simulink model "faultdetectioninagrid"  (R2021a)
settings: Solver=VariableStepAuto  StartTime=0.0  StopTime=10.0  RelTol=1e-3
libraries: spsMosfetLib x20, spsSeriesRLCBranchLib x16, spsVoltageMeasurementLib x13, spsCurrentMeasurementLib x10, spsPiSectionLineLib x10, pid_lib x9, spsGroundLib x6, spsMeanLib x5, simulink x5, spsACVoltageSourceLib x4, spsPLLLib x4, spsDiodeLib x1
settings Model: Creator=Himanik Panchal  LastModifiedBy=Himanik Panchal

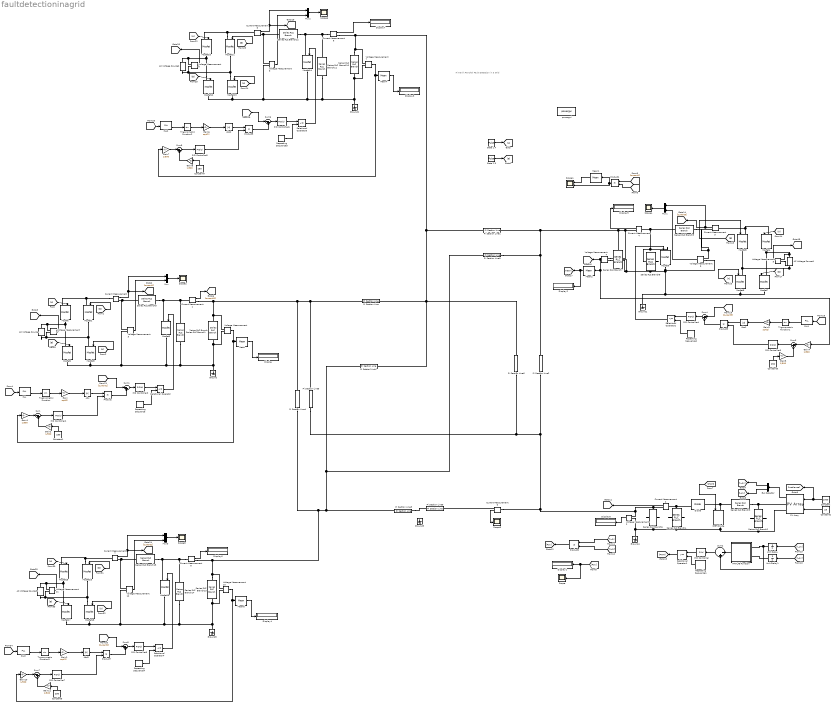
== system faultdetectioninagrid ==
  note: Himanik Panchal
      | Fault Detection in a Grid
  AC Voltage Source{,1..3} (4 alike) : spsACVoltageSourceLib/AC Voltage Source  Amplitude=230*sqrt(2)  Phase=0  Frequency=50  SampleTime=0  Measurements=None  BusType=swing  Pref=10e3  Qref=0  Qmin=-inf  Qmax=+inf
  Abs{,1..3} (4 alike) : Abs
  Bus Selector : BusSelector  OutputSignals=V_PV,I_PV
  Constant : Constant  Value=1000
  Constant{1,3..5} (4 alike) : Constant  Value=250
  Constant2 : Constant  Value=25
  Current Measurement{,1..9} (10 alike) : spsCurrentMeasurementLib/Current Measurement  PhasorSimulation=off  OutputType=Complex  PSBequivalent=0
  Diode : spsDiodeLib/Diode  Ron=0.001  Lon=0  Vf=0.8  IC=0  UseSnubber=0  Rs=500  Cs=250e-9  Measurements=on
  Display{,1..8} (9 alike) : Display
  Gain{,3,6,9} (4 alike) : Gain  Gain=sqrt(2)
  Gain{1..2,4..5,7..8,10..11} (8 alike) : Gain  Gain=1/500
  Gate 1,4 : DiscretePulseGenerator  PulseType=Time based  Period=0.02  PulseWidth=5  PhaseDelay=0.0033
  Gate 2,3 : DiscretePulseGenerator  PulseType=Time based  Period=0.02  PulseWidth=5  PhaseDelay=0.0033 + 0.01
  Ground{,1..5} (6 alike) : spsGroundLib/Ground  LConnTagsString=a
  IGBT/Diode : spsIGBTDiodeLib/IGBT//Diode  Ron=1e-3  Rs=1e5  Cs=inf  Measurements=on
  MATLAB Function : MATLAB Function  TreatAsAtomicUnit=on
  Mean{,1..2,4,6} (5 alike) : spsMeanLib/Mean  Freq=60  Vinit=0  Ts=0
  Mosfet{,1..19} (20 alike) : spsMosfetLib/Mosfet  Ron=0.1  Lon=0  Rd=0.01  Vfd=0  IC=0  Rs=1e5  Cs=inf  Measurements=off
  Mux{,1..3} (4 alike) : Mux  Inputs=2
  PID Controller : pid_lib/PID Controller  Controller=PI  Form=Parallel  TimeDomain=Continuous-time  UseExternalTs=off  SampleTime=-1  IntegratorMethod=Forward Euler  FilterMethod=Forward Euler  ControllerParametersSource=internal  P=.001  I=.01  D=0  UseFilter=on  N=100  TunerSelectOption=Transfer Function Based (PID Tuner App)  InitialConditionSource=internal  InitialConditionForIntegrator=0  InitialConditionForFilter=0  DifferentiatorICPrevScaledInput=0  ExternalReset=none  TrackingMode=off  Kt=1  LimitOutput=on  SatLimitsSource=internal  UpperSaturationLimit=.95  LowerSaturationLimit=0  LinearizeAsGain=on  AntiWindupMode=none  Kb=1  POutMin=[]  POutMax=[]  IOutMin=[]  IOutMax=[]  DOutMin=[]  DOutMax=[]  NOutMin=[]  NOutMax=[]  SumOutMin=[]  SumOutMax=[]  SaturationOutMin=[]  SaturationOutMax=[]  PParamMin=[]  PParamMax=[]  IParamMin=[]  IParamMax=[]  DParamMin=[]  DParamMax=[]  NParamMin=[]  NParamMax=[]  KbParamMin=[]  KbParamMax=[]  KtParamMin=[]  KtParamMax=[]  KbOutMin=[]  KbOutMax=[]  KtOutMin=[]  KtOutMax=[]  IntegratorOutMin=[]  IntegratorOutMax=[]  FilterOutMin=[]  FilterOutMax=[]  SumI1OutMin=[]  SumI1OutMax=[]  SumI2OutMin=[]  SumI2OutMax=[]  SumI3OutMin=[]  SumI3OutMax=[]  SumI4OutMin=[]  SumI4OutMax=[]  SumDOutMin=[]  SumDOutMax=[]  DifferentiatorOutMin=[]  DifferentiatorOutMax=[]  FilterDiffOutCoefMin=[]  FilterDiffOutCoefMax=[]  ReciprocalOutMin=[]  ReciprocalOutMax=[]  SumDenOutMin=[]  SumDenOutMax=[]  SumNumOutMin=[]  SumNumOutMax=[]  DivideOutMin=[]  DivideOutMax=[]  UdiffTsProdOutMin=[]  UdiffTsProdOutMax=[]  NTsProdOutMin=[]  NTsProdOutMax=[]  UintegralTsProdOutMin=[]  UintegralTsProdOutMax=[]  UngainTsProdOutMin=[]  UngainTsProdOutMax=[]  IntegratorContinuousStateAttributes=''  IntegratorStateMustResolveToSignalObject=off  IntegratorRTWStateStorageClass=Auto  FilterContinuousStateAttributes=''  FilterStateMustResolveToSignalObject=off  FilterRTWStateStorageClass=Auto  ParallelPVariant=InternalParameters  IdealPVariant=Disabled  IVariant=InternalParameters  DVariant=Disabled  IntegratorVariant=Continuous  SatVariant=Enabled  AWVariant=Passthrough  PCopyVariant=Disabled  TRVariant=Disabled  FdbkBlocksVariant=Forward  IdealPFdbkVariant=Disabled  SatFdbkVariant=Disabled  DerivativeFilterVariant=Disabled  NVariant=Disabled  NCopyVariant=Disabled_SignalSpec  FilterICVariant=Disabled  IntegratorICVariant=InternalICs  ExternalResetVariant=Disabled  TRSumVariant=Passthrough  SumFdbkVariant=Disabled  SumVariant=Sum_PI  TsampFilterVariant=InternalTs  TsampNgainVariant=Passthrough  TsampIntegralVariant=Passthrough  ExternalSaturationOutDataTypeStr=Inherit: Same as second input
  PID Controller{1..8} (8 alike) : pid_lib/PID Controller  Controller=PID  Form=Parallel  TimeDomain=Continuous-time  UseExternalTs=off  SampleTime=-1  IntegratorMethod=Forward Euler  FilterMethod=Forward Euler  ControllerParametersSource=internal  P=0.001  I=10  D=0  UseFilter=on  N=100  TunerSelectOption=Transfer Function Based (PID Tuner App)  InitialConditionSource=internal  InitialConditionForIntegrator=0  InitialConditionForFilter=0  DifferentiatorICPrevScaledInput=0  ExternalReset=none  TrackingMode=off  Kt=1  LimitOutput=off  SatLimitsSource=internal  UpperSaturationLimit=inf  LowerSaturationLimit=-inf  LinearizeAsGain=on  AntiWindupMode=none  Kb=1  POutMin=[]  POutMax=[]  IOutMin=[]  IOutMax=[]  DOutMin=[]  DOutMax=[]  NOutMin=[]  NOutMax=[]  SumOutMin=[]  SumOutMax=[]  SaturationOutMin=[]  SaturationOutMax=[]  PParamMin=[]  PParamMax=[]  IParamMin=[]  IParamMax=[]  DParamMin=[]  DParamMax=[]  NParamMin=[]  NParamMax=[]  KbParamMin=[]  KbParamMax=[]  KtParamMin=[]  KtParamMax=[]  KbOutMin=[]  KbOutMax=[]  KtOutMin=[]  KtOutMax=[]  IntegratorOutMin=[]  IntegratorOutMax=[]  FilterOutMin=[]  FilterOutMax=[]  SumI1OutMin=[]  SumI1OutMax=[]  SumI2OutMin=[]  SumI2OutMax=[]  SumI3OutMin=[]  SumI3OutMax=[]  SumI4OutMin=[]  SumI4OutMax=[]  SumDOutMin=[]  SumDOutMax=[]  DifferentiatorOutMin=[]  DifferentiatorOutMax=[]  FilterDiffOutCoefMin=[]  FilterDiffOutCoefMax=[]  ReciprocalOutMin=[]  ReciprocalOutMax=[]  SumDenOutMin=[]  SumDenOutMax=[]  SumNumOutMin=[]  SumNumOutMax=[]  DivideOutMin=[]  DivideOutMax=[]  UdiffTsProdOutMin=[]  UdiffTsProdOutMax=[]  NTsProdOutMin=[]  NTsProdOutMax=[]  UintegralTsProdOutMin=[]  UintegralTsProdOutMax=[]  UngainTsProdOutMin=[]  UngainTsProdOutMax=[]  IntegratorContinuousStateAttributes=''  IntegratorStateMustResolveToSignalObject=off  IntegratorRTWStateStorageClass=Auto  FilterContinuousStateAttributes=''  FilterStateMustResolveToSignalObject=off  FilterRTWStateStorageClass=Auto  ParallelPVariant=InternalParameters  IdealPVariant=Disabled  IVariant=InternalParameters  DVariant=InternalParameters  IntegratorVariant=Continuous  SatVariant=Disabled  AWVariant=Passthrough  PCopyVariant=Disabled  TRVariant=Disabled  FdbkBlocksVariant=Forward  IdealPFdbkVariant=Disabled  SatFdbkVariant=Disabled  DerivativeFilterVariant=ContFilter  NVariant=InternalParameters  NCopyVariant=Disabled  FilterICVariant=InternalICsFilter  IntegratorICVariant=InternalICs  ExternalResetVariant=Disabled  TRSumVariant=Passthrough  SumFdbkVariant=Disabled  SumVariant=Sum_PID  TsampFilterVariant=InternalTs  TsampNgainVariant=Passthrough  TsampIntegralVariant=Passthrough  ExternalSaturationOutDataTypeStr=Inherit: Same as second input
  PLL{,1..3} (4 alike) : spsPLLLib/PLL  Fmin=45  Par_Init=[0, 60]  ParK=[180, 3200, 1]  TcD=1e-4  MaxRateChangeFreq=12  FilterCutOffFreq=25  Ts=0  AGC=on
      settings: SourceProductBaseCode=PS
  PV Array : spsPVArrayLib/PV Array  Npar=47  Nser=10  PlotType=array @ 25 deg.C & specified irradiances  S_vec="[ 1000  500  100 ]"  Temp_C_vec="[ 45 25  ]"  ModuleName=User-defined  PlotWhenSelected=off  Pm=213.15  Ncell=60  Voc=36.3  Isc=7.84  Vm=29  Im=7.35  beta_Voc_pc=-0.36099  alpha_Isc_pc=0.102  beta_Voc=-0.13104  alpha_Isc=0.0079968  IL=7.8654  I0=2.9273e-10  nI=0.98119  Rsh=313.0553  Rs=0.39381  RobustModel=off  RobustCellTemperature=313.3991  BAL=on  Tc=1e-6  Tfilter=5e-5
  Pi Section Line : spsPiSectionLineLib/Pi Section Line  LConnTagsString=1  RConnTagsString=1  Phases=1  PiSections=1  Length=0.75  Frequency=60  Resistance=0.12  Inductance=300e-6  Capacitance=0.5e-6  Measurements=None  Measurements2=None
      settings: SourceProductBaseCode=PS
  Pi Section Line1 : spsPiSectionLineLib/Pi Section Line  LConnTagsString=1  RConnTagsString=1  Phases=1  PiSections=1  Length=0.8  Frequency=60  Resistance=0.12  Inductance=300e-6  Capacitance=0.5e-6  Measurements=None  Measurements2=None
      settings: SourceProductBaseCode=PS
  Pi Section Line2 : spsPiSectionLineLib/Pi Section Line  LConnTagsString=1  RConnTagsString=1  Phases=1  PiSections=1  Length=1.2  Frequency=60  Resistance=0.12  Inductance=300e-6  Capacitance=0.5e-6  Measurements=None  Measurements2=None
      settings: SourceProductBaseCode=PS
  Pi Section Line3 : spsPiSectionLineLib/Pi Section Line  LConnTagsString=1  RConnTagsString=1  Phases=1  PiSections=1  Length=0.5  Frequency=60  Resistance=0.12  Inductance=300e-6  Capacitance=0.5e-6  Measurements=None  Measurements2=None
      settings: SourceProductBaseCode=PS
  Pi Section Line4 : spsPiSectionLineLib/Pi Section Line  LConnTagsString=1  RConnTagsString=1  Phases=1  PiSections=1  Length=0.8  Frequency=60  Resistance=0.12  Inductance=300e-6  Capacitance=0.5e-6  Measurements=None  Measurements2=None
      settings: SourceProductBaseCode=PS
  Pi Section Line5 : spsPiSectionLineLib/Pi Section Line  LConnTagsString=1  RConnTagsString=1  Phases=1  PiSections=1  Length=1.1  Frequency=60  Resistance=0.12  Inductance=300e-6  Capacitance=0.5e-6  Measurements=None  Measurements2=None
      settings: SourceProductBaseCode=PS
  Pi Section Line6 : spsPiSectionLineLib/Pi Section Line  LConnTagsString=1  RConnTagsString=1  Phases=1  PiSections=1  Length=0.8  Frequency=60  Resistance=0.12  Inductance=300e-6  Capacitance=0.5e-6  Measurements=None  Measurements2=None
      settings: SourceProductBaseCode=PS
  Pi Section Line7 : spsPiSectionLineLib/Pi Section Line  LConnTagsString=1  RConnTagsString=1  Phases=1  PiSections=1  Length=1  Frequency=60  Resistance=0.12  Inductance=300e-6  Capacitance=0.5e-6  Measurements=None  Measurements2=None
      settings: SourceProductBaseCode=PS
  Pi Section Line8 : spsPiSectionLineLib/Pi Section Line  LConnTagsString=1  RConnTagsString=1  Phases=1  PiSections=1  Length=1.2  Frequency=60  Resistance=0.12  Inductance=300e-6  Capacitance=0.5e-6  Measurements=None  Measurements2=None
      settings: SourceProductBaseCode=PS
  Pi Section Line9 : spsPiSectionLineLib/Pi Section Line  LConnTagsString=1  RConnTagsString=1  Phases=1  PiSections=1  Length=0.5  Frequency=60  Resistance=0.12  Inductance=300e-6  Capacitance=0.5e-6  Measurements=None  Measurements2=None
      settings: SourceProductBaseCode=PS
  Product{,1..3,5,7} (6 alike) : Product
  Relational Operator{,2..4} (4 alike) : RelationalOperator  Operator=<=  OutDataTypeStr=boolean  RndMeth=Simplest
  Relational Operator1 : RelationalOperator  OutDataTypeStr=boolean  RndMeth=Simplest
  Repeating Sequence{,2..4} (4 alike) : simulink/Sources/Repeating Sequence  rep_seq_t=[0 0.5 1]/100  rep_seq_y=[0 1 0]
  Repeating Sequence1 : simulink/Sources/Repeating Sequence  rep_seq_t=[0 0.0002]  rep_seq_y=[0 1]
  Scope{,2..4,6,8} (6 alike) : Scope
  Scope1 : Scope  NumInputPorts=2
  Series RLC Branch{,7,10,13} (4 alike) : spsSeriesRLCBranchLib/Series RLC Branch  LConnTagsString=__new0  RConnTagsString=__new0  BranchType=R  Resistance=120  Inductance=1e-3  SetiL0=off  InitialCurrent=0  Capacitance=1e-6  Setx0=off  InitialVoltage=0  Measurements=None
  Series RLC Branch{1,8,11,14} (4 alike) : spsSeriesRLCBranchLib/Series RLC Branch  LConnTagsString=__new0  RConnTagsString=__new0  BranchType=C  Resistance=20  Inductance=1e-3  SetiL0=off  InitialCurrent=0  Capacitance=1e-6  Setx0=off  InitialVoltage=0  Measurements=None
  Series RLC Branch{5,9,12,15} (4 alike) : spsSeriesRLCBranchLib/Series RLC Branch  LConnTagsString=__new0  RConnTagsString=__new0  BranchType=L  Resistance=20  Inductance=1e-3  SetiL0=off  InitialCurrent=0  Capacitance=1e-6  Setx0=off  InitialVoltage=0  Measurements=None
  Series RLC Branch2 : spsSeriesRLCBranchLib/Series RLC Branch  LConnTagsString=__new0  RConnTagsString=__new0  BranchType=RC  Resistance=1e-4  Inductance=1e-3  SetiL0=off  InitialCurrent=0  Capacitance=100e-6  Setx0=off  InitialVoltage=0  Measurements=None
  Series RLC Branch3 : spsSeriesRLCBranchLib/Series RLC Branch  LConnTagsString=__new0  RConnTagsString=__new0  BranchType=L  Resistance=.1  Inductance=1.45e-3  SetiL0=off  InitialCurrent=0  Capacitance=100e-6  Setx0=off  InitialVoltage=0  Measurements=None
  Series RLC Branch4 : spsSeriesRLCBranchLib/Series RLC Branch  LConnTagsString=__new0  RConnTagsString=__new0  BranchType=C  Resistance=1e-4  Inductance=1e-3  SetiL0=off  InitialCurrent=0  Capacitance=322e-6  Setx0=off  InitialVoltage=0  Measurements=None
  Series RLC Branch6 : spsSeriesRLCBranchLib/Series RLC Branch  LConnTagsString=__new0  RConnTagsString=__new0  BranchType=R  Resistance=2  Inductance=1e-3  SetiL0=off  InitialCurrent=0  Capacitance=33e-6  Setx0=off  InitialVoltage=0  Measurements=None
  Sum{,1..8} (9 alike) : Sum  Inputs=|-+
  Trigonometric Function{,1..3} (4 alike) : Trigonometry
  Unit Delay : UnitDelay  SampleTime=-1  HasFrameUpgradeWarning=on
  Unit Delay1 : UnitDelay  SampleTime=-1  HasFrameUpgradeWarning=on
  Voltage Measurement{,1..12} (13 alike) : spsVoltageMeasurementLib/Voltage Measurement  PhasorSimulation=off  OutputType=Complex  PSBequivalent=0
  powergui : spspowerguiLib/powergui  Priority=1  SimulationMode=Continuous  SampleTime=50e-6  frequency=60  Iterations=50  frequencyindice=50  Pbase=100e6  ErrMax=1e-4  UnitsV=kV  UnitsW=MW  buscounter=0  FunctionMessages=off  echomessages=off  EnableUseOfTLC=off  CurrentSourceSwitches=off  DisableSnubberDevices=off  DisableRonSwitches=off  DisableVfSwitches=off  DisplayEquations=off  AutomaticDiscreteSolvers=off  SolverType=Tustin/Backward Euler (TBE)  Interpol=off  ExternalGateDelay=off  methode=off  Ts=100  x0status=blocks  SPID=on  SwTol=0  HookPort=off  NonlinearTolerance=1e-4  nMaxIteration=100  ContinueOnMaxIteration=off  RestoreLinks=warning  ResistiveCurrentMeasurement=off  Frange=[0:2:500]  Ylog=off  Xlog=on  ShowGrid=off  save=off  variable=ZData  structure=0  ZoomFFT=off  StartTime=0.0  cycles=1  DisplayStyle=1  fundamental=60  FreqAxis=off  MaxFrequency=1000  frequencyindicesteady=1  RmsSteady=1  display=off
  wires:
  Trigonometric Function/1 -> Gain/1
  Gain1/1 -> Sum/1
  [A] -> Mosfet/1
  Voltage Measurement/1 -> Mean/1, Gain1/1
  Gain2/1 -> Sum/2
  PLL/2 -> Trigonometric Function/1
  Sum/1 -> PID Controller1/1
  Current Measurement/1 -> Mux/1, [current1]
  [B] -> Mosfet1/1
  [InputV] -> PLL/1
  Voltage Measurement1/1 -> [InputV1]
  Relational Operator/1 -> Mosfet6/1
  Repeating Sequence/1 -> Relational Operator/2
  Abs/1 -> Product/1
  Mux/1 -> Scope2/1
  Constant1/1 -> Gain2/1
  Sum1/1 -> PID Controller2/1
  Gate 2,3/1 -> [B]
  Product/1 -> Sum1/2
  [B] -> Mosfet2/1
  PID Controller2/1 -> Relational Operator/1
  Mean/1 -> Display/1
  [A] -> Mosfet3/1
  PID Controller1/1 -> Product/2
  Voltage Measurement3/1 -> Mux/2
  Gate 1,4/1 -> [A]
  [current1] -> Sum1/1
  Gain/1 -> Abs/1
  Current Measurement1/1 -> [current11]
  [current1] -> Product1/1
  [OutputV] -> Product1/2
  Product1/1 -> Mean1/1, Scope1/2
  Current Measurement2/1 -> [iboost]
  [Ppv] -> Scope/1, Display1/1
  [i_pv] -> Unit Delay1/1
  PV Array/1 -> Bus Selector/1
  Bus Selector/2 -> [i_pv]  "<I_PV>"
  Unit Delay1/1 -> MATLAB Function/2(I)
  Unit Delay/1 -> MATLAB Function/1(V), Sum2/2
  Product2/1 -> [Ppv]
  Sum2/1 -> PID Controller/1
  MATLAB Function/1(Vref) -> Sum2/1
  [i_pv] -> Product2/2
  [v_pv] -> Product2/1
  Repeating Sequence1/1 -> Relational Operator1/2
  [v_pv] -> Unit Delay/1
  [PWM] -> IGBT/Diode/1
  Constant/1 -> PV Array/1, [Irradiance]
  Bus Selector/1 -> [v_pv]  "<V_PV>"
  Relational Operator1/1 -> [PWM]
  Constant2/1 -> PV Array/2
  PID Controller/1 -> Relational Operator1/1
  Gain3/1 -> Abs1/1
  [current3] -> Sum4/1
  Voltage Measurement6/1 -> Mux1/2
  PID Controller3/1 -> Product3/2
  [A] -> Mosfet8/1
  Mean2/1 -> [mean], Display2/1
  PID Controller4/1 -> Relational Operator2/1
  [B] -> Mosfet7/1
  Product3/1 -> Sum4/2
  Sum4/1 -> PID Controller4/1
  Constant3/1 -> Gain5/1
  Mux1/1 -> Scope4/1
  Abs1/1 -> Product3/1
  Repeating Sequence2/1 -> Relational Operator2/2
  Relational Operator2/1 -> Mosfet9/1
  Voltage Measurement5/1 -> [InputV3]
  [InputV] -> PLL1/1
  [B] -> Mosfet5/1
  Current Measurement3/1 -> [current3], Mux1/1
  Sum3/1 -> PID Controller3/1
  PLL1/2 -> Trigonometric Function1/1
  Gain5/1 -> Sum3/2
  Voltage Measurement4/1 -> [OutputV], Gain4/1, Mean2/1
  [A] -> Mosfet4/1
  Gain4/1 -> Sum3/1
  Trigonometric Function1/1 -> Gain3/1
  [A] -> Mosfet13/1
  Mux2/1 -> Scope6/1
  Voltage Measurement8/1 -> [InputV]
  Sum5/1 -> PID Controller5/1
  Repeating Sequence3/1 -> Relational Operator3/2
  [A] -> Mosfet10/1
  [current] -> Sum6/1
  [B] -> Mosfet12/1
  Product5/1 -> Sum6/2
  Gain6/1 -> Abs2/1
  Constant4/1 -> Gain8/1
  Voltage Measurement9/1 -> Mux2/2
  Relational Operator3/1 -> Mosfet14/1
  Voltage Measurement7/1 -> Mean4/1, Gain7/1
  PID Controller6/1 -> Relational Operator3/1
  [InputV] -> PLL2/1
  Abs2/1 -> Product5/1
  Sum6/1 -> PID Controller6/1
  Gain8/1 -> Sum5/2
  Gain7/1 -> Sum5/1
  Trigonometric Function2/1 -> Gain6/1
  [B] -> Mosfet11/1
  Current Measurement5/1 -> Mux2/1, [current]
  PID Controller5/1 -> Product5/2
  PLL2/2 -> Trigonometric Function2/1
  Mean4/1 -> Display3/1
  [A] -> Mosfet18/1
  Mux3/1 -> Scope8/1
  Voltage Measurement11/1 -> [InputV2]
  Sum7/1 -> PID Controller7/1
  Repeating Sequence4/1 -> Relational Operator4/2
  [A] -> Mosfet15/1
  [current2] -> Sum8/1
  [B] -> Mosfet17/1
  Product7/1 -> Sum8/2
  Gain9/1 -> Abs3/1
  Constant5/1 -> Gain11/1
  Voltage Measurement12/1 -> Mux3/2
  Relational Operator4/1 -> Mosfet19/1
  Voltage Measurement10/1 -> Mean6/1, Gain10/1
  PID Controller8/1 -> Relational Operator4/1
  [InputV] -> PLL3/1
  Abs3/1 -> Product7/1
  Sum8/1 -> PID Controller8/1
  Gain11/1 -> Sum7/2
  Gain10/1 -> Sum7/1
  Trigonometric Function3/1 -> Gain9/1
  [B] -> Mosfet16/1
  Current Measurement7/1 -> Mux3/1, [current2]
  PID Controller7/1 -> Product7/2
  PLL3/2 -> Trigonometric Function3/1
  Mean6/1 -> Display4/1
  Mean1/1 -> Scope1/1
  Current Measurement4/1 -> Display5/1
  Current Measurement8/1 -> Display6/1
  Current Measurement6/1 -> Display7/1
  Voltage Measurement2/1 -> Display8/1
  Current Measurement9/1 -> Scope3/1
  connections:
  Mosfet6/RConn1 -- Voltage Measurement3/LConn2 -- Mosfet2/RConn1 -- Mosfet3/RConn1 -- Ground/LConn1 -- Voltage Measurement/LConn2 -- Series RLC Branch/RConn1 -- Series RLC Branch1/RConn1
  Current Measurement/RConn1 -- Series RLC Branch5/RConn1 -- Voltage Measurement3/LConn1
  AC Voltage Source/LConn1 -- Voltage Measurement1/LConn2 -- Mosfet1/RConn1 -- Mosfet3/LConn1
  Series RLC Branch5/LConn1 -- Mosfet6/LConn1 -- Series RLC Branch1/LConn1 -- Current Measurement1/LConn1
  Current Measurement/LConn1 -- Mosfet/LConn1 -- Mosfet1/LConn1
  AC Voltage Source/RConn1 -- Voltage Measurement1/LConn1 -- Mosfet/RConn1 -- Mosfet2/LConn1
  Voltage Measurement/LConn1 -- Current Measurement1/RConn1 -- Pi Section Line4/LConn1 -- Pi Section Line/LConn1 -- Pi Section Line5/LConn1 -- Series RLC Branch/LConn1
  Diode/LConn1 -- IGBT/Diode/LConn1 -- Series RLC Branch3/LConn1
  Series RLC Branch3/RConn1 -- PV Array/RConn1 -- Series RLC Branch2/LConn1
  Current Measurement2/RConn1 -- Series RLC Branch6/LConn1 -- Pi Section Line5/RConn1 -- Pi Section Line6/RConn1 -- Pi Section Line2/RConn1 -- Current Measurement9/LConn1 -- Voltage Measurement2/LConn1
  Current Measurement2/LConn1 -- Series RLC Branch4/LConn1 -- Diode/RConn1
  Series RLC Branch4/RConn1 -- Series RLC Branch2/RConn1 -- PV Array/RConn2 -- IGBT/Diode/RConn1 -- Ground4/LConn1 -- Voltage Measurement2/LConn2 -- Series RLC Branch6/RConn1
  Mosfet9/RConn1 -- Voltage Measurement4/LConn2 -- Series RLC Branch7/RConn1 -- Series RLC Branch8/RConn1 -- Ground1/LConn1 -- Mosfet7/RConn1 -- Mosfet8/RConn1 -- Voltage Measurement6/LConn2
  Series RLC Branch9/RConn1 -- Voltage Measurement6/LConn1 -- Current Measurement3/RConn1
  AC Voltage Source1/LConn1 -- Mosfet5/RConn1 -- Mosfet8/LConn1 -- Voltage Measurement5/LConn2
  Series RLC Branch9/LConn1 -- Series RLC Branch8/LConn1 -- Mosfet9/LConn1 -- Current Measurement4/LConn1
  Mosfet4/LConn1 -- Mosfet5/LConn1 -- Current Measurement3/LConn1
  AC Voltage Source1/RConn1 -- Mosfet4/RConn1 -- Mosfet7/LConn1 -- Voltage Measurement5/LConn1
  Voltage Measurement4/LConn1 -- Current Measurement4/RConn1 -- Series RLC Branch7/LConn1 -- Pi Section Line1/RConn1 -- Pi Section Line2/LConn1 -- Pi Section Line8/RConn1
  Series RLC Branch10/LConn1 -- Current Measurement6/RConn1 -- Pi Section Line6/LConn1 -- Pi Section Line7/RConn1 -- Pi Section Line/RConn1 -- Pi Section Line1/LConn1 -- Voltage Measurement7/LConn1
  Mosfet12/LConn1 -- AC Voltage Source2/RConn1 -- Voltage Measurement8/LConn1 -- Mosfet10/RConn1
  Mosfet13/RConn1 -- Mosfet12/RConn1 -- Voltage Measurement9/LConn2 -- Mosfet14/RConn1 -- Ground2/LConn1 -- Voltage Measurement7/LConn2 -- Series RLC Branch10/RConn1 -- Series RLC Branch11/RConn1
  Mosfet11/LConn1 -- Mosfet10/LConn1 -- Current Measurement5/LConn1
  Mosfet13/LConn1 -- Mosfet11/RConn1 -- AC Voltage Source2/LConn1 -- Voltage Measurement8/LConn2
  Current Measurement6/LConn1 -- Series RLC Branch11/LConn1 -- Series RLC Branch12/LConn1 -- Mosfet14/LConn1
  Current Measurement5/RConn1 -- Series RLC Branch12/RConn1 -- Voltage Measurement9/LConn1
  Series RLC Branch13/LConn1 -- Current Measurement8/RConn1 -- Pi Section Line3/RConn1 -- Pi Section Line7/LConn1 -- Pi Section Line8/LConn1 -- Pi Section Line4/RConn1 -- Voltage Measurement10/LConn1
  Mosfet17/LConn1 -- AC Voltage Source3/RConn1 -- Voltage Measurement11/LConn1 -- Mosfet15/RConn1
  Mosfet18/RConn1 -- Mosfet17/RConn1 -- Voltage Measurement12/LConn2 -- Mosfet19/RConn1 -- Ground3/LConn1 -- Voltage Measurement10/LConn2 -- Series RLC Branch13/RConn1 -- Series RLC Branch14/RConn1
  Mosfet16/LConn1 -- Mosfet15/LConn1 -- Current Measurement7/LConn1
  Mosfet18/LConn1 -- Mosfet16/RConn1 -- AC Voltage Source3/LConn1 -- Voltage Measurement11/LConn2
  Current Measurement8/LConn1 -- Series RLC Branch14/LConn1 -- Series RLC Branch15/LConn1 -- Mosfet19/LConn1
  Current Measurement7/RConn1 -- Series RLC Branch15/RConn1 -- Voltage Measurement12/LConn1
  Current Measurement9/RConn1 -- Pi Section Line9/LConn1
  Pi Section Line3/LConn1 -- Pi Section Line9/RConn1

== matlab function faultdetectioninagrid/MATLAB Function ==
  data: V input; Vref output; I input
function Vref = RefGen(V, I)

Vrefmax = 363;
Vrefmin = 0;
Vrefinit = 300;
deltaVref = 1;
persistent Vold Pold Vrefold;

dataType = 'double';

if isempty(Vold)
Vold = 0;
Pold = 0;
Vrefold = Vrefinit;
end

P = V*I;
dV = V-Vold;
dP = P-Pold;

if dP ~= 0
    if dP<0
        if dV<0
            Vref = Vrefold + deltaVref;
        else
            Vref = Vrefold - deltaVref;
        end
    else
        if dV<0
            Vref = Vrefold - deltaVref;
        else
            Vref = Vrefold + deltaVref;
        end
    end
else
    Vref = Vrefold;
end

if Vref >= Vrefmax | Vref <= Vrefmin
    Vref = Vrefold;
end

Vrefold = Vref;
Vold = V;
Pold = P;
